simulink model "Assignment_model"  (R2017a)
settings: Solver=ode45  StartTime=0.0  StopTime=200  RelTol=1e-3  EnableMultiTasking=on
settings Model: Creator=Administrator  LastModifiedBy=sarthakbhagat
settings DataIOCC: LimitDataPoints=on  SaveFormat=Array
settings OptimizationCC: LifeSpan=inf
settings DebuggingCC: SolverPrmCheckMsg=warning  AllowSymbolicDim=off  SFUnexpectedBacktrackingDiag=warning  SFNoUnconditionalDefaultTransitionDiag=warning  SFExecutionAtInitializationDiag=none
settings HardwareCC: ProdBitPerPointer=32  ProdBitPerSizeT=32  ProdBitPerPtrDiffT=32  ProdLargestAtomicFloat=None  ProdIntDivRoundTo=Undefined  ProdEndianess=Unspecified  ProdWordSize=32  ProdHWDeviceType=32-bit Generic
settings ModelReferenceCC: PropagateSignalLabelsOutOfModel=off
settings GRTTargetCC: TargetLangStandard=C89/C90 (ANSI)  GeneratePreprocessorConditionals=Disable all
settings ConfigComp: CovMetricSettings=dw  CovHtmlReporting=on  CovSaveCumulativeToWorkspaceVar=on  CovSaveSingleToWorkspaceVar=on  CovExternalEMLEnable=off  CovSFcnEnable=off

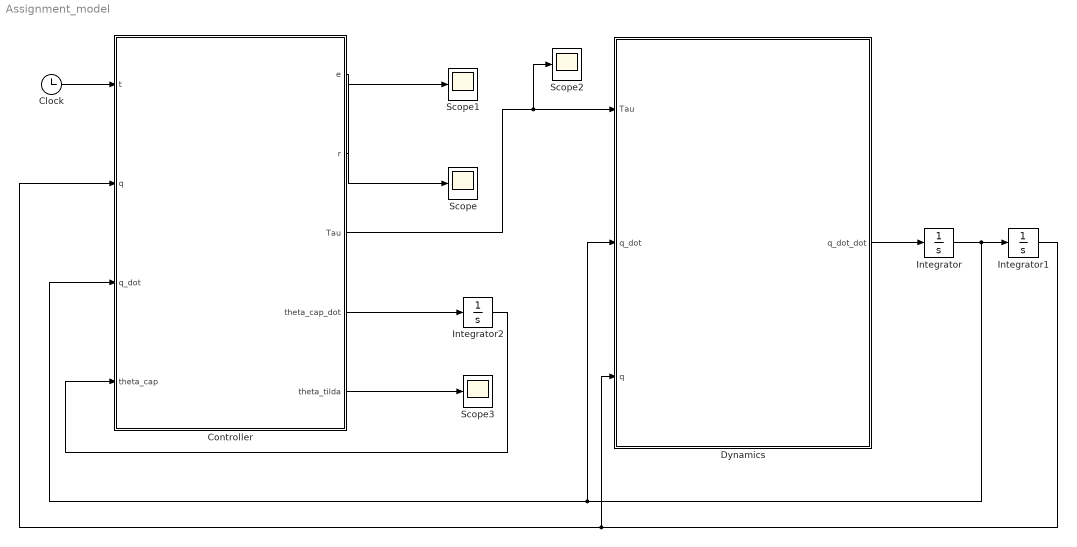
== system Assignment_model ==
  Clock : Clock
      settings: Decimation=50
  Controller : MATLAB Function  TreatAsAtomicUnit=on
  Dynamics : MATLAB Function  TreatAsAtomicUnit=on
  Integrator : Integrator  InitialCondition=[1;-1]
  Integrator1 : Integrator  InitialCondition=[1,1]
  Integrator2 : Integrator  InitialCondition=[1;1;1;1;1]
  Scope{,1..3} (4 alike) : Scope
  wires:
  Dynamics/1(q_dot_dot) -> Integrator/1
  Integrator/1 -> Dynamics/2(q_dot), Controller/3(q_dot), Integrator1/1
  Integrator1/1 -> Controller/2(q), Dynamics/3(q)
  Controller/3(Tau) -> Scope2/1, Dynamics/1(Tau)
  Clock/1 -> Controller/1(t)
  Controller/1(e) -> Scope/1
  Controller/2(r) -> Scope1/1
  Controller/4(theta_cap_dot) -> Integrator2/1
  Integrator2/1 -> Controller/4(theta_cap)
  Controller/5(theta_tilda) -> Scope3/1

== matlab function Assignment_model/Controller ==
  data: e output; r output; Tau output; t input; q input; q_dot input; theta_cap_dot output; theta_cap input; theta_tilda output
function [e,r,Tau,theta_cap_dot,theta_tilda] = controller(t,q,q_dot,theta_cap)

c2=cos(q(2));
s2=sin(q(2));
alpha=10;
k=10;
middle_coef = 10;
middle_matrix = middle_coef * eye(5);

theta = [3.473; 0.196; 0.242; 5.3; 1.1];

qd=[0.5*sin(t);2*cos(t/4)];
qd_dot=[0.5*cos(t);-0.5*sin(t/4)];
qd_ddot=[-0.5*sin(t);-0.25*cos(t/4)];
e=q-qd; 
e_dot=q_dot-qd_dot;

r=e_dot+alpha*e; 

z1 = [0 0 2*s2*q_dot(1)*q_dot(2)+s2*q_dot(2)*q_dot(2) 0 0; 
      0 0 -s2*q_dot(1)*q_dot(1) 0 0];

z2 = -[0 0 0 -q_dot(1) 0;
       0 0 0 0 -q_dot(2)];
   
z3 = [0 0 -s2*q_dot(1)*r(2)-s2*q_dot(2)*r(2)-s2*q_dot(1)*r(1) 0 0; 
      0 0 s2*q_dot(1)*r(1) 0 0];
  
z4 = -[qd_ddot(1) qd_ddot(2) 2*c2*qd_ddot(1)+c2*qd_ddot(2) 0 0;
      0 qd_ddot(1)+qd_ddot(2) c2*qd_ddot(1) 0 0];
  
z5 = alpha*[e_dot(1) e_dot(2) 2*c2*e_dot(1)+c2*e_dot(2) 0 0;
            0 e_dot(1)+e_dot(2) c2*e_dot(1) 0 0];

Z = z1+z2+z3+z4+z5;

Tau = -Z*theta_cap - k*r - e;
theta_tilda = theta - theta_cap;
theta_cap_dot = middle_matrix*transpose(Z)*r;

== matlab function Assignment_model/Dynamics ==
  data: Tau input; q_dot_dot output; q_dot input; q input
function q_dot_dot   = dynamics(Tau,q_dot,q)
%#codegen
%p1 = theta_cap(1);
%p2 = theta_cap(2);
%p3 = theta_cap(3);
%fd1 = theta_cap(4);
%fd2 = theta_cap(5);

p1 = 3.473; 
p2 = 0.196; 
p3 = 0.242; 
fd1 = 5.3; 
fd2 = 1.1;

c2=cos(q(2));
s2=sin(q(2));
% alpha=1;

M=[p1+2*p3*c2 p2+p3*c2;p2+p3*c2 p2];% Inertia matrix
Vm=[-p3*s2*q_dot(2) -p3*s2*(q_dot(1)+q_dot(2));p3*s2*q_dot(1) 0];%Centripetal coriolis matrix
fd=[fd1 0;0 fd2]; % Friction matrix
q_dot_dot=-M\(Vm*q_dot+fd*q_dot-Tau);   %EL dynamics
